simulink model "modelo"  (R2025a)
settings: Solver=VariableStepAuto  StartTime=0.0  StopTime=10.0  RelTol=1e-3
libraries: cstblocks x4
settings Model: Creator=joaof  LastModifiedBy=joaof

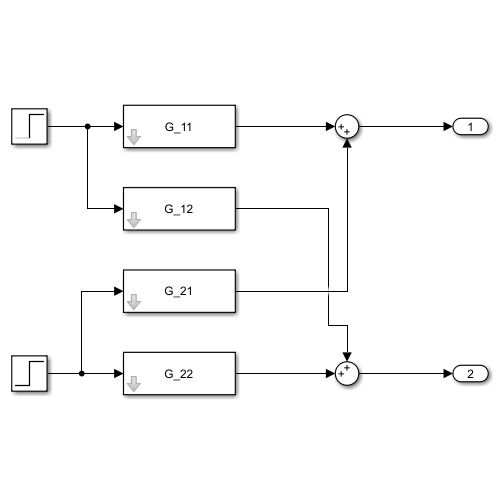
[thumbnail: Simulink's stored preview of the top-level diagram]
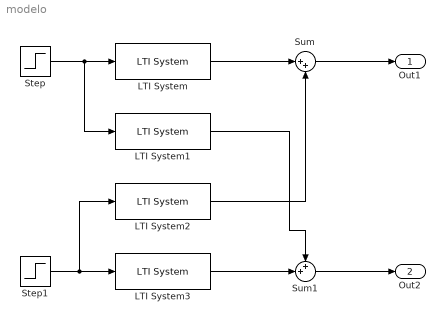
== system modelo ==
  LTI System : cstblocks/LTI System  sys=G_11  IC=[]  PadeOrder=0
  LTI System1 : cstblocks/LTI System  sys=G_12  IC=[]  PadeOrder=0
  LTI System2 : cstblocks/LTI System  sys=G_21  IC=[]  PadeOrder=0
  LTI System3 : cstblocks/LTI System  sys=G_22  IC=[]  PadeOrder=0
  Step : Step  SampleTime=0
  Step1 : Step  SampleTime=0
  Sum : Sum  Inputs=|++
  Sum1 : Sum  Inputs=++|
  Out1 : Outport
  Out2 : Outport  Port=2
  wires:
  Step1/1 -> LTI System2/1, LTI System3/1
  Step/1 -> LTI System1/1, LTI System/1
  LTI System3/1 -> Sum1/2
  LTI System/1 -> Sum/1
  Sum/1 -> Out1/1
  LTI System2/1 -> Sum/2
  LTI System1/1 -> Sum1/1
  Sum1/1 -> Out2/1
